simulink model "gtm_aeromodel"  (Simulink 7.2)
settings: Solver=ode45  StartTime=0.0  StopTime=10.0  RelTol=1e-3
undefined symbols (not defined in the file or in its folder): A_BLCG, A_BW, A_CW, A_FSCG, A_FSREF_in, A_SW, A_WLCG, A_WLREF, ALPHA0, bclowb, bclowbx_FMACH, bcmowb, bcmowbx_FHP, bcmowby_FMACH, cda, cdax_FLPDEF, cddr, cddrx_FMACH, cdo, cdox_FLPDEF, cdt1, cdt1x_mach, cdt2, cdt2x_mach, cdto, cdtox_mach, cdwb, cdwbx_FALPHA, cdwby_FMACH, clat, clatfr, clatfrx_FHP, clatfry_FMACH, clatx_mach, clawbfr, clawbfrx_FHP, clawbfry_FMACH, cldefr, cldefrx_FHP, cldefry_FMACH, cldtab, cldtabx_FMACH, clqwb, clqwbfr, clqwbfrx_FHP, clqwbfry_FMACH, clqwbx_mach, cltdd, cltddx_FHP, cltddy_FMACH, clwb, clwbtdd, clwbtddx_FHP, clwbtddy_FMACH, clwbx_FALPHA, clwby_FMACH, clwbzdd, clwbzddx_FHP, clwbzddy_FMACH, clzdd ... (+196)
libraries: model_lib x1
(part 4 of 10)

== system gtm_aeromodel/get aero forces and moments/AERODYNAMICS/Force  Coefficients/DRAG /bcddf ==
  flap : Inport  OutDataType=sfix(16)  OutScaling=2^0
  Logical Operator : Logic
  Logical Operator1 : Logic
  Product1 : Product  Inputs=3  OutDataType=sfix(16)  OutScaling=2^0  SaturateOnIntegerOverflow=on  RndMeth=Zero  InputSameDT=on  OutDataTypeStr=Inherit: Same as first input
  Product2 : Product  Inputs=3  OutDataType=sfix(16)  OutScaling=2^0  SaturateOnIntegerOverflow=on  RndMeth=Zero  InputSameDT=on  OutDataTypeStr=Inherit: Same as first input
  Relational Operator : RelationalOperator  Operator=>  InputSameDT=on
  Relational Operator1 : RelationalOperator  Operator=<=  InputSameDT=on
  Relational Operator2 : RelationalOperator  Operator=>  InputSameDT=on
  Relational Operator3 : RelationalOperator  Operator=<=  InputSameDT=on
  Relational Operator4 : RelationalOperator  Operator=>  InputSameDT=on
  Sum : Sum  Inputs=+++  OutDataType=sfix(16)  OutScaling=2^0  SaturateOnIntegerOverflow=on  InputSameDT=on  OutDataTypeStr=Inherit: Same as first input
  Sum2 : Sum  OutDataType=sfix(16)  OutScaling=2^0  SaturateOnIntegerOverflow=on  InputSameDT=on  OutDataTypeStr=Inherit: Same as first input
  Sum{3..5,8} (4 alike) : Sum  Inputs=-+  OutDataType=sfix(16)  OutScaling=2^0  SaturateOnIntegerOverflow=on  InputSameDT=on  OutDataTypeStr=Inherit: Same as first input
  Sum6 : Sum  OutDataType=sfix(16)  OutScaling=2^0  SaturateOnIntegerOverflow=on  InputSameDT=on  OutDataTypeStr=Inherit: Same as first input
  Switch5 : Switch  Threshold=0.5  SaturateOnIntegerOverflow=on  InputSameDT=on
  Switch6 : Switch  Threshold=0.5  SaturateOnIntegerOverflow=on  InputSameDT=on
  Switch7 : Switch  Threshold=0.5  SaturateOnIntegerOverflow=on  InputSameDT=on
  zero : Constant  Value=0  OutDataType=sfix(16)  OutScaling=2^0
  zero1 : Constant  Value=10  OutDataType=sfix(16)  OutScaling=2^0
  zero11 : Constant  Value=-0.01  OutDataType=sfix(16)  OutScaling=2^0
  zero12 : Constant  Value=-0.013  OutDataType=sfix(16)  OutScaling=2^0
  zero13 : Constant  Value=-0.0175  OutDataType=sfix(16)  OutScaling=2^0
  zero2 : Constant  Value=0  OutDataType=sfix(16)  OutScaling=2^0
  zero5 : Constant  Value=20  OutDataType=sfix(16)  OutScaling=2^0
  zero6 : Constant  Value=10  OutDataType=sfix(16)  OutScaling=2^0
  zero7 : Constant  Value=0.1  OutDataType=sfix(16)  OutScaling=2^0
  zero8 : Constant  Value=20  OutDataType=sfix(16)  OutScaling=2^0
  zero9 : Constant  Value=1/19  OutDataType=sfix(16)  OutScaling=2^0
  bcddf : Outport  OutDataType=sfix(16)  OutScaling=2^0  InitialOutput=0
  wires:
  Sum6/1 -> Switch7/1
  zero9/1 -> Product2/2
  Sum5/1 -> Product2/3
  zero8/1 -> Sum5/1
  Sum2/1 -> Switch6/1
  Switch7/1 -> Sum/3
  Switch6/1 -> Sum/2
  Switch5/1 -> Sum/1
  Relational Operator4/1 -> Switch7/2
  zero5/1 -> Relational Operator4/2, Relational Operator3/2
  Sum/1 -> bcddf/1
  zero2/1 -> Switch7/3, Switch6/3, Switch5/3
  Logical Operator1/1 -> Switch6/2
  Relational Operator3/1 -> Logical Operator1/2
  Relational Operator2/1 -> Logical Operator1/1
  zero1/1 -> Relational Operator2/2, Relational Operator1/2
  zero/1 -> Relational Operator/2
  Logical Operator/1 -> Switch5/2
  Relational Operator1/1 -> Logical Operator/2
  Relational Operator/1 -> Logical Operator/1
  Sum3/1 -> Product1/3
  zero6/1 -> Sum3/1
  flap/1 -> Sum5/2, Relational Operator4/1, Relational Operator3/1, Relational Operator2/1, Relational Operator1/1, Relational Operator/1, Sum3/2
  zero11/1 -> Switch5/1, Sum2/1, Sum4/1
  Sum4/1 -> Product1/1
  Product1/1 -> Sum2/2
  zero12/1 -> Sum4/2, Sum8/1, Sum6/1
  zero13/1 -> Sum8/2
  zero7/1 -> Product1/2
  Sum8/1 -> Product2/1
  Product2/1 -> Sum6/2

== system gtm_aeromodel/get aero forces and moments/AERODYNAMICS/Force  Coefficients/DRAG /bcdwb ==
  clwb : Inport  OutDataType=sfix(16)  OutScaling=2^0
  Product6 : Product  OutDataType=sfix(16)  OutScaling=2^0  SaturateOnIntegerOverflow=on  RndMeth=Zero  InputSameDT=on  OutDataTypeStr=Inherit: Same as first input
  bcwb : Sum  Inputs=-+  OutDataType=sfix(16)  OutScaling=2^0  SaturateOnIntegerOverflow=on  InputSameDT=on  OutDataTypeStr=Inherit: Same as first input
  bcwb_FC8 : Constant  Value=.003  OutDataType=sfix(16)  OutScaling=2^0
  bcwb_FC9 : Constant  Value=.023  OutDataType=sfix(16)  OutScaling=2^0
  bcdwb_ : Outport  OutDataType=sfix(16)  OutScaling=2^0  InitialOutput=0
  wires:
  bcwb_FC8/1 -> bcwb/1
  clwb/1 -> Product6/1
  bcwb_FC9/1 -> Product6/2
  Product6/1 -> bcwb/2
  bcwb/1 -> bcdwb_/1

== system gtm_aeromodel/get aero forces and moments/AERODYNAMICS/Force  Coefficients/LIFT/CLDETAB ==
  mach : Inport  OutDataType=sfix(16)  OutScaling=2^0
  eletab : Inport  Port=2  OutDataType=sfix(16)  OutScaling=2^0
  Product : Product  OutDataType=sfix(16)  OutScaling=2^0  SaturateOnIntegerOverflow=on  RndMeth=Zero  InputSameDT=on  OutDataTypeStr=Inherit: Same as first input
  cldetab_ : Subsystem  mask(1-D Table){z=cldtabx_FMACH, tab=cldtab}
      mask prompts: z "Z vector:"; tab "Table:"
      mask help: 1-D Table Look Up. Enter monotonic Z vector amd table. See the help for more info.
      mask Help: The Z vector must be monotonic.  Z indexes into the columns of the 1-D tables.   Table does not extrapolate beyound the break vectors
      mask Display: plot(@2)
  cldetab : Outport  OutDataType=sfix(16)  OutScaling=2^0  InitialOutput=0
  wires:
  cldetab_/1(Interp Value) -> Product/1
  Product/1 -> cldetab/1
  eletab/1 -> Product/2
  mach/1 -> cldetab_/1(Z)

== system gtm_aeromodel/get aero forces and moments/AERODYNAMICS/Force  Coefficients/LIFT/CLGE ==
  hob : Inport  OutDataType=sfix(16)  OutScaling=2^0
  alpha : Inport  Port=2  OutDataType=sfix(16)  OutScaling=2^0
  flap : Inport  Port=3  OutDataType=sfix(16)  OutScaling=2^0
  dclhob : Subsystem  mask(1-2-3 Table){@1=dclhobx_HOB, @2=dclhoby_FALPHA, @3=dclhobz_FLPDEF, @4=dclhob}
      mask prompts: @1 "X vector:"; @2 "Y vector:"; @3 "Z vector:"; @4 "Table:"
      mask help: 3-D Table Look Up. Enter monotonic X, Y and Z vectors and a matrix of 2-D tables. See the help for more info.
      mask init:
      | x=@1;y=@2;z=@3;tab=@4;
      mask Help: The X, Y and Z vectors must be monotonic.   The 3-D table is a horizontal concatenation of  2-D tables.  X  indexes into the columns of the 2-D tables & Y indexes into the rows of the 2-D tables.  Z indexes into the table levels (starting with the 1st 2-D table).   The input values are x, y and z respectively (e.g., top port = x).
      mask Display: plot([0 2 2 0 0],[0 0 2 2 0],[0 2 2.9 0.95 0],[2 2 2.7 2.7 2],[2 2.9 2.9 2 2],[0 0.85 2.7 2 0])
  cdge : Outport  OutDataType=sfix(16)  OutScaling=2^0  InitialOutput=0
  wires:
  dclhob/1(Interp Value) -> cdge/1
  hob/1 -> dclhob/1(X)
  alpha/1 -> dclhob/2(Y)
  flap/1 -> dclhob/3(Z)

== system gtm_aeromodel/get aero forces and moments/AERODYNAMICS/Force  Coefficients/LIFT/CLQWB ==
  note: fqsv=q*cbar/2vt
  mach : Inport  OutDataType=sfix(16)  OutScaling=2^0
  Q' : Inport  Port=2  OutDataType=sfix(16)  OutScaling=2^0
  flex : Inport  Port=3  OutDataType=sfix(16)  OutScaling=2^0
  altitude : Inport  Port=4  OutDataType=sfix(16)  OutScaling=2^0
  Product : Product  Inputs=3  OutDataType=sfix(16)  OutScaling=2^0  SaturateOnIntegerOverflow=on  RndMeth=Zero  InputSameDT=on  OutDataTypeStr=Inherit: Same as first input
  Switch5 : Switch  Threshold=0.5  SaturateOnIntegerOverflow=on  InputSameDT=on
  clqwb_ : Subsystem  mask(1-D Table){z=clqwbx_mach, tab=clqwb}
      mask prompts: z "Z vector:"; tab "Table:"
      mask help: 1-D Table Look Up. Enter monotonic Z vector amd table. See the help for more info.
      mask Help: The Z vector must be monotonic.  Z indexes into the columns of the 1-D tables.   Table does not extrapolate beyound the break vectors
      mask Display: plot(@2)
  clqwbfr : Subsystem  TreatAsAtomicUnit=on
  one : Constant  Value=1.0  OutDataType=sfix(16)  OutScaling=2^0
  clq : Outport  OutDataType=sfix(16)  OutScaling=2^0  InitialOutput=0
  wires:
  clqwb_/1(Interp Value) -> Product/1
  mach/1 -> clqwbfr/2(mach1), clqwb_/1(Z)
  altitude/1 -> clqwbfr/1(altitude)
  Switch5/1 -> Product/3
  one/1 -> Switch5/3
  flex/1 -> Switch5/2, clqwbfr/Enable
  clqwbfr/1(clqwbfr) -> Switch5/1
  Q'/1 -> Product/2
  Product/1 -> clq/1

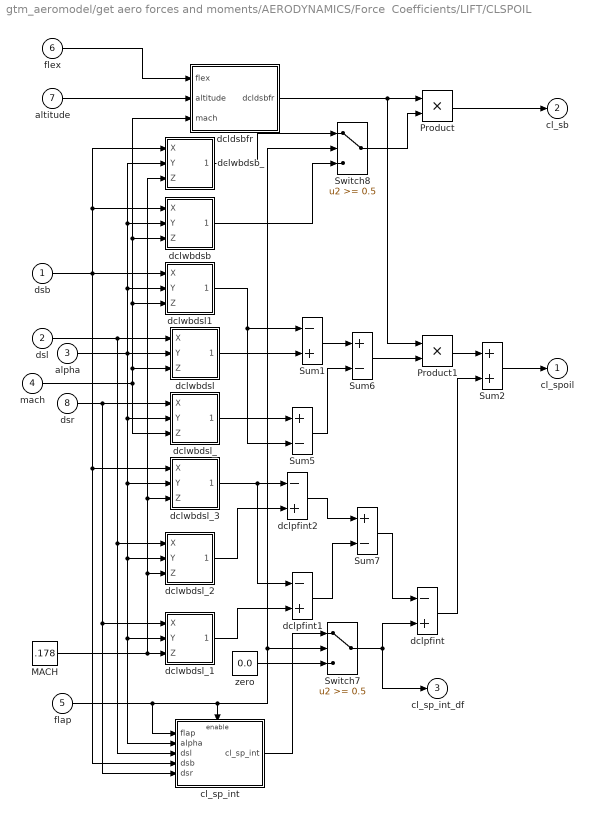
== system gtm_aeromodel/get aero forces and moments/AERODYNAMICS/Force  Coefficients/LIFT/CLSPOIL ==
  dsb : Inport  OutDataType=sfix(16)  OutScaling=2^0
  dsl : Inport  Port=2  OutDataType=sfix(16)  OutScaling=2^0
  alpha : Inport  Port=3  OutDataType=sfix(16)  OutScaling=2^0
  mach : Inport  Port=4  OutDataType=sfix(16)  OutScaling=2^0
  flap : Inport  Port=5  OutDataType=sfix(16)  OutScaling=2^0
  flex : Inport  Port=6  OutDataType=sfix(16)  OutScaling=2^0
  altitude : Inport  Port=7  OutDataType=sfix(16)  OutScaling=2^0
  dsr : Inport  Port=8  OutDataType=sfix(16)  OutScaling=2^0
  MACH : Constant  Value=.178  OutDataType=sfix(16)  OutScaling=2^0
  Product : Product  OutDataType=sfix(16)  OutScaling=2^0  SaturateOnIntegerOverflow=on  RndMeth=Zero  InputSameDT=on  OutDataTypeStr=Inherit: Same as first input
  Product1 : Product  OutDataType=sfix(16)  OutScaling=2^0  SaturateOnIntegerOverflow=on  RndMeth=Zero  InputSameDT=on  OutDataTypeStr=Inherit: Same as first input
  Sum1 : Sum  Inputs=-+  OutDataType=sfix(16)  OutScaling=2^0  SaturateOnIntegerOverflow=on  InputSameDT=on  OutDataTypeStr=Inherit: Same as first input
  Sum2 : Sum  OutDataType=sfix(16)  OutScaling=2^0  SaturateOnIntegerOverflow=on  InputSameDT=on  OutDataTypeStr=Inherit: Same as first input
  Sum5 : Sum  Inputs=+-  OutDataType=sfix(16)  OutScaling=2^0  SaturateOnIntegerOverflow=on  InputSameDT=on  OutDataTypeStr=Inherit: Same as first input
  Sum6 : Sum  Inputs=+-  OutDataType=sfix(16)  OutScaling=2^0  SaturateOnIntegerOverflow=on  InputSameDT=on  OutDataTypeStr=Inherit: Same as first input
  Sum7 : Sum  Inputs=+-  OutDataType=sfix(16)  OutScaling=2^0  SaturateOnIntegerOverflow=on  InputSameDT=on  OutDataTypeStr=Inherit: Same as first input
  Switch7 : Switch  Threshold=0.5  SaturateOnIntegerOverflow=on  InputSameDT=on
  Switch8 : Switch  Threshold=0.5  SaturateOnIntegerOverflow=on  InputSameDT=on
  cl_sp_int : Subsystem  TreatAsAtomicUnit=on
  dcldsbfr : Subsystem
  dclpfint : Sum  Inputs=-+  OutDataType=sfix(16)  OutScaling=2^0  SaturateOnIntegerOverflow=on  InputSameDT=on  OutDataTypeStr=Inherit: Same as first input
  dclpfint1 : Sum  Inputs=-+  OutDataType=sfix(16)  OutScaling=2^0  SaturateOnIntegerOverflow=on  InputSameDT=on  OutDataTypeStr=Inherit: Same as first input
  dclpfint2 : Sum  Inputs=-+  OutDataType=sfix(16)  OutScaling=2^0  SaturateOnIntegerOverflow=on  InputSameDT=on  OutDataTypeStr=Inherit: Same as first input
  dclwbdsb : Subsystem  mask(1-2-3 Table){@1=dclwbdsbx_DSB, @2=dclwbdsby_ALPHA, @3=dclwbdsbz_FMACH, @4=dclwbdsb}
      mask prompts: @1 "X vector:"; @2 "Y vector:"; @3 "Z vector:"; @4 "Table:"
      mask help: 3-D Table Look Up. Enter monotonic X, Y and Z vectors and a matrix of 2-D tables. See the help for more info.
      mask init:
      | x=@1;y=@2;z=@3;tab=@4;
      mask Help: The X, Y and Z vectors must be monotonic.   The 3-D table is a horizontal concatenation of  2-D tables.  X  indexes into the columns of the 2-D tables & Y indexes into the rows of the 2-D tables.  Z indexes into the table levels (starting with the 1st 2-D table).   The input values are x, y and z respectively (e.g., top port = x).
      mask Display: plot([0 2 2 0 0],[0 0 2 2 0],[0 2 2.9 0.95 0],[2 2 2.7 2.7 2],[2 2.9 2.9 2 2],[0 0.85 2.7 2 0])
  dclwbdsb_ : Subsystem  mask(1-2-3 Table){@1=dclwbdsbx_DSB, @2=dclwbdsby_ALPHA, @3=dclwbdsbz_FMACH, @4=dclwbdsb}
      mask prompts: @1 "X vector:"; @2 "Y vector:"; @3 "Z vector:"; @4 "Table:"
      mask help: 3-D Table Look Up. Enter monotonic X, Y and Z vectors and a matrix of 2-D tables. See the help for more info.
      mask init:
      | x=@1;y=@2;z=@3;tab=@4;
      mask Help: The X, Y and Z vectors must be monotonic.   The 3-D table is a horizontal concatenation of  2-D tables.  X  indexes into the columns of the 2-D tables & Y indexes into the rows of the 2-D tables.  Z indexes into the table levels (starting with the 1st 2-D table).   The input values are x, y and z respectively (e.g., top port = x).
      mask Display: plot([0 2 2 0 0],[0 0 2 2 0],[0 2 2.9 0.95 0],[2 2 2.7 2.7 2],[2 2.9 2.9 2 2],[0 0.85 2.7 2 0])
  dclwbdsl : Subsystem  mask(1-2-3 Table){@1=dclwbdslx_DSL, @2=dclwbdsly_FALPHA, @3=dclwbdslz_FMACH, @4=dclwbdsl}
      mask prompts: @1 "X vector:"; @2 "Y vector:"; @3 "Z vector:"; @4 "Table:"
      mask help: 3-D Table Look Up. Enter monotonic X, Y and Z vectors and a matrix of 2-D tables. See the help for more info.
      mask init:
      | x=@1;y=@2;z=@3;tab=@4;
      mask Help: The X, Y and Z vectors must be monotonic.   The 3-D table is a horizontal concatenation of  2-D tables.  X  indexes into the columns of the 2-D tables & Y indexes into the rows of the 2-D tables.  Z indexes into the table levels (starting with the 1st 2-D table).   The input values are x, y and z respectively (e.g., top port = x).
      mask Display: plot([0 2 2 0 0],[0 0 2 2 0],[0 2 2.9 0.95 0],[2 2 2.7 2.7 2],[2 2.9 2.9 2 2],[0 0.85 2.7 2 0])
  dclwbdsl1 : Subsystem  mask(1-2-3 Table){@1=dclwbdslx_DSL, @2=dclwbdsly_FALPHA, @3=dclwbdslz_FMACH, @4=dclwbdsl}
      mask prompts: @1 "X vector:"; @2 "Y vector:"; @3 "Z vector:"; @4 "Table:"
      mask help: 3-D Table Look Up. Enter monotonic X, Y and Z vectors and a matrix of 2-D tables. See the help for more info.
      mask init:
      | x=@1;y=@2;z=@3;tab=@4;
      mask Help: The X, Y and Z vectors must be monotonic.   The 3-D table is a horizontal concatenation of  2-D tables.  X  indexes into the columns of the 2-D tables & Y indexes into the rows of the 2-D tables.  Z indexes into the table levels (starting with the 1st 2-D table).   The input values are x, y and z respectively (e.g., top port = x).
      mask Display: plot([0 2 2 0 0],[0 0 2 2 0],[0 2 2.9 0.95 0],[2 2 2.7 2.7 2],[2 2.9 2.9 2 2],[0 0.85 2.7 2 0])
  dclwbdsl_ : Subsystem  mask(1-2-3 Table){@1=dclwbdslx_DSL, @2=dclwbdsly_FALPHA, @3=dclwbdslz_FMACH, @4=dclwbdsl}
      mask prompts: @1 "X vector:"; @2 "Y vector:"; @3 "Z vector:"; @4 "Table:"
      mask help: 3-D Table Look Up. Enter monotonic X, Y and Z vectors and a matrix of 2-D tables. See the help for more info.
      mask init:
      | x=@1;y=@2;z=@3;tab=@4;
      mask Help: The X, Y and Z vectors must be monotonic.   The 3-D table is a horizontal concatenation of  2-D tables.  X  indexes into the columns of the 2-D tables & Y indexes into the rows of the 2-D tables.  Z indexes into the table levels (starting with the 1st 2-D table).   The input values are x, y and z respectively (e.g., top port = x).
      mask Display: plot([0 2 2 0 0],[0 0 2 2 0],[0 2 2.9 0.95 0],[2 2 2.7 2.7 2],[2 2.9 2.9 2 2],[0 0.85 2.7 2 0])
  dclwbdsl_1 : Subsystem  mask(1-2-3 Table){@1=dclwbdslx_DSL, @2=dclwbdsly_FALPHA, @3=dclwbdslz_FMACH, @4=dclwbdsl}
      mask prompts: @1 "X vector:"; @2 "Y vector:"; @3 "Z vector:"; @4 "Table:"
      mask help: 3-D Table Look Up. Enter monotonic X, Y and Z vectors and a matrix of 2-D tables. See the help for more info.
      mask init:
      | x=@1;y=@2;z=@3;tab=@4;
      mask Help: The X, Y and Z vectors must be monotonic.   The 3-D table is a horizontal concatenation of  2-D tables.  X  indexes into the columns of the 2-D tables & Y indexes into the rows of the 2-D tables.  Z indexes into the table levels (starting with the 1st 2-D table).   The input values are x, y and z respectively (e.g., top port = x).
      mask Display: plot([0 2 2 0 0],[0 0 2 2 0],[0 2 2.9 0.95 0],[2 2 2.7 2.7 2],[2 2.9 2.9 2 2],[0 0.85 2.7 2 0])
  dclwbdsl_2 : Subsystem  mask(1-2-3 Table){@1=dclwbdslx_DSL, @2=dclwbdsly_FALPHA, @3=dclwbdslz_FMACH, @4=dclwbdsl}
      mask prompts: @1 "X vector:"; @2 "Y vector:"; @3 "Z vector:"; @4 "Table:"
      mask help: 3-D Table Look Up. Enter monotonic X, Y and Z vectors and a matrix of 2-D tables. See the help for more info.
      mask init:
      | x=@1;y=@2;z=@3;tab=@4;
      mask Help: The X, Y and Z vectors must be monotonic.   The 3-D table is a horizontal concatenation of  2-D tables.  X  indexes into the columns of the 2-D tables & Y indexes into the rows of the 2-D tables.  Z indexes into the table levels (starting with the 1st 2-D table).   The input values are x, y and z respectively (e.g., top port = x).
      mask Display: plot([0 2 2 0 0],[0 0 2 2 0],[0 2 2.9 0.95 0],[2 2 2.7 2.7 2],[2 2.9 2.9 2 2],[0 0.85 2.7 2 0])
  dclwbdsl_3 : Subsystem  mask(1-2-3 Table){@1=dclwbdslx_DSL, @2=dclwbdsly_FALPHA, @3=dclwbdslz_FMACH, @4=dclwbdsl}
      mask prompts: @1 "X vector:"; @2 "Y vector:"; @3 "Z vector:"; @4 "Table:"
      mask help: 3-D Table Look Up. Enter monotonic X, Y and Z vectors and a matrix of 2-D tables. See the help for more info.
      mask init:
      | x=@1;y=@2;z=@3;tab=@4;
      mask Help: The X, Y and Z vectors must be monotonic.   The 3-D table is a horizontal concatenation of  2-D tables.  X  indexes into the columns of the 2-D tables & Y indexes into the rows of the 2-D tables.  Z indexes into the table levels (starting with the 1st 2-D table).   The input values are x, y and z respectively (e.g., top port = x).
      mask Display: plot([0 2 2 0 0],[0 0 2 2 0],[0 2 2.9 0.95 0],[2 2 2.7 2.7 2],[2 2.9 2.9 2 2],[0 0.85 2.7 2 0])
  zero : Constant  Value=0.0  OutDataType=sfix(16)  OutScaling=2^0
  cl_spoil : Outport  OutDataType=sfix(16)  OutScaling=2^0  InitialOutput=0
  cl_sb : Outport  Port=2  OutDataType=sfix(16)  OutScaling=2^0  InitialOutput=0
  cl_sp_int_df : Outport  Port=3  OutDataType=sfix(16)  OutScaling=2^0  InitialOutput=0
  wires:
  flex/1 -> dcldsbfr/1(flex)
  dclwbdsb_/1(Interp Value) -> Switch8/1
  dclwbdsb/1(Interp Value) -> Switch8/3
  dclwbdsl1/1(Interp Value) -> Sum5/2, Sum1/1
  MACH/1 -> dclwbdsb_/3(Z), dclwbdsl_3/3(Z), dclwbdsl_2/3(Z), dclwbdsl_1/3(Z)
  Sum7/1 -> dclpfint/1
  dclpfint1/1 -> Sum7/2
  dclpfint2/1 -> Sum7/1
  dclwbdsl_2/1(Interp Value) -> dclpfint2/2
  dclwbdsl_3/1(Interp Value) -> dclpfint2/1, dclpfint1/1
  dclwbdsl_1/1(Interp Value) -> dclpfint1/2
  dsr/1 -> cl_sp_int/5(dsr), dclwbdsl_1/1(X), dclwbdsl_/1(X)
  mach/1 -> dclwbdsl_/3(Z), dclwbdsb/3(Z), dcldsbfr/3(mach), dclwbdsl1/3(Z), dclwbdsl/3(Z)
  dclwbdsl/1(Interp Value) -> Sum1/2
  alpha/1 -> dclwbdsl_2/2(Y), dclwbdsl_1/2(Y), cl_sp_int/2(alpha), dclwbdsl_3/2(Y), dclwbdsl_/2(Y), dclwbdsl/2(Y), dclwbdsl1/2(Y), dclwbdsb/2(Y), dclwbdsb_/2(Y)
  dsl/1 -> dclwbdsl_2/1(X), cl_sp_int/3(dsl), dclwbdsl/1(X)
  Sum6/1 -> Product1/2
  Sum5/1 -> Sum6/2
  Sum1/1 -> Sum6/1
  dclwbdsl_/1(Interp Value) -> Sum5/1
  dclpfint/1 -> Sum2/2
  Product1/1 -> Sum2/1
  Sum2/1 -> cl_spoil/1
  flap/1 -> cl_sp_int/1(flap), Switch8/2, Switch7/2, cl_sp_int/Enable
  cl_sp_int/1(cl_sp_int) -> Switch7/1
  zero/1 -> Switch7/3
  dsb/1 -> dclwbdsb_/1(X), dclwbdsb/1(X), dclwbdsl_3/1(X), cl_sp_int/4(dsb), dclwbdsl1/1(X)
  dcldsbfr/1(dcldsbfr) -> Product1/1, Product/1
  Product/1 -> cl_sb/1
  Switch8/1 -> Product/2
  altitude/1 -> dcldsbfr/2(altitude)
  Switch7/1 -> dclpfint/2, cl_sp_int_df/1

== system gtm_aeromodel/get aero forces and moments/AERODYNAMICS/Force  Coefficients/LIFT/CLTP ==
  mach : Inport  OutDataType=sfix(16)  OutScaling=2^0
  alphat : Inport  Port=2  OutDataType=sfix(16)  OutScaling=2^0
  altitude : Inport  Port=3  OutDataType=sfix(16)  OutScaling=2^0
  norm acc g's : Inport  Port=4  OutDataType=sfix(16)  OutScaling=2^0
  qdot : Inport  Port=5  OutDataType=sfix(16)  OutScaling=2^0
  flex : Inport  Port=6  OutDataType=sfix(16)  OutScaling=2^0
  Product1 : Product  OutDataType=sfix(16)  OutScaling=2^0  SaturateOnIntegerOverflow=on  RndMeth=Zero  InputSameDT=on  OutDataTypeStr=Inherit: Same as first input
  Product2 : Product  OutDataType=sfix(16)  OutScaling=2^0  SaturateOnIntegerOverflow=on  RndMeth=Zero  InputSameDT=on  OutDataTypeStr=Inherit: Same as first input
  Switch6 : Switch  Threshold=0.5  SaturateOnIntegerOverflow=on  InputSameDT=on
  Switch7 : Switch  Threshold=0.5  SaturateOnIntegerOverflow=on  InputSameDT=on
  clat : Subsystem  mask(1-D Table){z=clatx_mach, tab=clat}
      mask prompts: z "Z vector:"; tab "Table:"
      mask help: 1-D Table Look Up. Enter monotonic Z vector amd table. See the help for more info.
      mask Help: The Z vector must be monotonic.  Z indexes into the columns of the 1-D tables.   Table does not extrapolate beyound the break vectors
      mask Display: plot(@2)
  cltailflx : Subsystem  TreatAsAtomicUnit=on
  one : Constant  OutDataType=sfix(16)  OutScaling=2^0
  zero : Constant  Value=0.0  OutDataType=sfix(16)  OutScaling=2^0
  cltp : Outport  OutDataType=sfix(16)  OutScaling=2^0  InitialOutput=0
  cltfr : Outport  Port=2  OutDataType=sfix(16)  OutScaling=2^0  InitialOutput=0
  wires:
  clat/1(Interp Value) -> Product1/1
  Switch7/1 -> Product1/2
  Product1/1 -> Product2/1
  alphat/1 -> Product2/2
  Product2/1 -> cltp/1
  one/1 -> Switch7/3
  cltailflx/2(clatfr) -> Switch7/1
  altitude/1 -> cltailflx/1(altitude)
  qdot/1 -> cltailflx/4(qdot)
  norm acc g's/1 -> cltailflx/3(norm acc g's)
  Switch6/1 -> cltfr/1
  cltailflx/1(cltflx) -> Switch6/1
  flex/1 -> Switch7/2, cltailflx/Enable, Switch6/2
  zero/1 -> Switch6/3
  mach/1 -> cltailflx/2(Mach), clat/1(Z)

== system gtm_aeromodel/get aero forces and moments/AERODYNAMICS/Force  Coefficients/LIFT/CLWB ==
  alpha : Inport  OutDataType=sfix(16)  OutScaling=2^0
  mach : Inport  Port=2  OutDataType=sfix(16)  OutScaling=2^0
  flap : Inport  Port=3  OutDataType=sfix(16)  OutScaling=2^0
  flex : Inport  Port=4  OutDataType=sfix(16)  OutScaling=2^0
  altitude : Inport  Port=5  OutDataType=sfix(16)  OutScaling=2^0
  qdyn : Inport  Port=6  OutDataType=sfix(16)  OutScaling=2^0
  norm acc g's : Inport  Port=7  OutDataType=sfix(16)  OutScaling=2^0
  qdot : Inport  Port=8  OutDataType=sfix(16)  OutScaling=2^0
  dsb : Inport  Port=9  OutDataType=sfix(16)  OutScaling=2^0
  CLWBFLEX : Subsystem  TreatAsAtomicUnit=on
  Product1 : Product  OutDataType=sfix(16)  OutScaling=2^0  SaturateOnIntegerOverflow=on  RndMeth=Zero  InputSameDT=on  OutDataTypeStr=Inherit: Same as first input
  Sum : Sum  OutDataType=sfix(16)  OutScaling=2^0  SaturateOnIntegerOverflow=on  InputSameDT=on  OutDataTypeStr=Inherit: Same as first input
  Sum2 : Sum  Inputs=+-  OutDataType=sfix(16)  OutScaling=2^0  SaturateOnIntegerOverflow=on  InputSameDT=on  OutDataTypeStr=Inherit: Same as first input
  Sum4 : Sum  OutDataType=sfix(16)  OutScaling=2^0  SaturateOnIntegerOverflow=on  InputSameDT=on  OutDataTypeStr=Inherit: Same as first input
  Switch{5..6,8,10} (4 alike) : Switch  Threshold=0.5  SaturateOnIntegerOverflow=on  InputSameDT=on
  cl_flap_ : Subsystem  TreatAsAtomicUnit=on
  clwb_ : Subsystem  mask(2-D Table){y=clwbx_FALPHA, z=clwby_FMACH, tab=clwb}
      mask prompts: y "Y vector:"; z "Z vector:"; tab "Table:"
      mask help: 2-D Table Look Up. Enter monotonic Y and Z vectors and a matrix of 2-D tables. See the help for more info.
      mask Help: The Y and Z vectors must be monotonic.  Y  indexes into the columns of the 2-D table & Z indexes into the rows of the 2-D tables.   The input values are y and z respectively (e.g., top port = y).
      mask Display: plot(-10,-10,110,110,[90,50,10],[90,40,30],[90,50,10],[50,26,20],[90,50,10],[22,13,10])
  clwb_zero : Subsystem  mask(2-D Table){y=clwbx_FALPHA, z=clwby_FMACH, tab=clwb}
      mask prompts: y "Y vector:"; z "Z vector:"; tab "Table:"
      mask help: 2-D Table Look Up. Enter monotonic Y and Z vectors and a matrix of 2-D tables. See the help for more info.
      mask Help: The Y and Z vectors must be monotonic.  Y  indexes into the columns of the 2-D table & Z indexes into the rows of the 2-D tables.   The input values are y and z respectively (e.g., top port = y).
      mask Display: plot(-10,-10,110,110,[90,50,10],[90,40,30],[90,50,10],[50,26,20],[90,50,10],[22,13,10])
  constant1 : Constant  Value=0.0  OutDataType=sfix(16)  OutScaling=2^0
  constant3 : Constant  Value=1.0  OutDataType=sfix(16)  OutScaling=2^0
  zero : Constant  Value=0.0  OutDataType=sfix(16)  OutScaling=2^0
  zero_ : Constant  Value=0.0  OutDataType=sfix(16)  OutScaling=2^0
  clwb : Outport  OutDataType=sfix(16)  OutScaling=2^0  InitialOutput=0
  cl_flap : Outport  Port=2  OutDataType=sfix(16)  OutScaling=2^0  InitialOutput=0
  dclsbfint : Outport  Port=3  OutDataType=sfix(16)  OutScaling=2^0  InitialOutput=0
  cl_flx : Outport  Port=4  OutDataType=sfix(16)  OutScaling=2^0  InitialOutput=0
  wires:
  CLWBFLEX/2(cl_flx) -> cl_flx/1
  CLWBFLEX/1(clawbfr) -> Switch8/1
  constant3/1 -> Switch8/3
  CLWBFLEX/3(fdclowb) -> Switch6/1
  Product1/1 -> Sum/2
  Sum4/1 -> Sum/1
  Switch10/1 -> dclsbfint/1
  cl_flap_/2(dclsbfint) -> Switch10/1
  dsb/1 -> cl_flap_/5(dsb)
  Switch8/1 -> Product1/2
  flex/1 -> cl_flap_/4(flex), Switch8/2, Switch6/2, CLWBFLEX/Enable
  qdot/1 -> CLWBFLEX/4(qdot)
  norm acc g's/1 -> CLWBFLEX/3(norm acc g's)
  clwb_zero/1(Interp Value) -> Sum2/2, Sum4/2
  zero/1 -> clwb_zero/1(Y)
  altitude/1 -> CLWBFLEX/1(altitude)
  constant1/1 -> Switch6/3
  qdyn/1 -> cl_flap_/3(qdyn)
  alpha/1 -> cl_flap_/2(alpha), clwb_/1(Y)
  mach/1 -> clwb_zero/2(Z), CLWBFLEX/2(Mach), clwb_/2(Z)
  cl_flap_/1(cl_flap) -> Switch5/1
  flap/1 -> cl_flap_/1(flap), cl_flap_/Enable, Switch5/2, Switch10/2
  zero_/1 -> Switch5/3, Switch10/3
  Switch6/1 -> Sum4/1
  clwb_/1(Interp Value) -> Sum2/1
  Sum2/1 -> Product1/1
  Switch5/1 -> cl_flap/1
  Sum/1 -> clwb/1

== system gtm_aeromodel/get aero forces and moments/AERODYNAMICS/Force  Coefficients/LIFT/DCLDE ==
  elev : Inport  OutDataType=sfix(16)  OutScaling=2^0
  alphat : Inport  Port=2  OutDataType=sfix(16)  OutScaling=2^0
  mach : Inport  Port=3  OutDataType=sfix(16)  OutScaling=2^0
  flex : Inport  Port=4  OutDataType=sfix(16)  OutScaling=2^0
  altitude : Inport  Port=5  OutDataType=sfix(16)  OutScaling=2^0
  Product : Product  OutDataType=sfix(16)  OutScaling=2^0  SaturateOnIntegerOverflow=on  RndMeth=Zero  InputSameDT=on  OutDataTypeStr=Inherit: Same as first input
  Switch5 : Switch  Threshold=0.5  SaturateOnIntegerOverflow=on  InputSameDT=on
  cldefr : Subsystem  TreatAsAtomicUnit=on
  constant3 : Constant  Value=1.0  OutDataType=sfix(16)  OutScaling=2^0
  dclde_ : Subsystem  mask(1-2-3 Table){@1=dcldex_FELE, @2=dcldey_ALPHAT, @3=dcldez_FMACH, @4=dclde}
      mask prompts: @1 "X vector:"; @2 "Y vector:"; @3 "Z vector:"; @4 "Table:"
      mask help: 3-D Table Look Up. Enter monotonic X, Y and Z vectors and a matrix of 2-D tables. See the help for more info.
      mask init:
      | x=@1;y=@2;z=@3;tab=@4;
      mask Help: The X, Y and Z vectors must be monotonic.   The 3-D table is a horizontal concatenation of  2-D tables.  X  indexes into the columns of the 2-D tables & Y indexes into the rows of the 2-D tables.  Z indexes into the table levels (starting with the 1st 2-D table).   The input values are x, y and z respectively (e.g., top port = x).
      mask Display: plot([0 2 2 0 0],[0 0 2 2 0],[0 2 2.9 0.95 0],[2 2 2.7 2.7 2],[2 2.9 2.9 2 2],[0 0.85 2.7 2 0])
  dclde : Outport  OutDataType=sfix(16)  OutScaling=2^0  InitialOutput=0
  wires:
  constant3/1 -> Switch5/3
  Switch5/1 -> Product/2
  Product/1 -> dclde/1
  dclde_/1(Interp Value) -> Product/1
  flex/1 -> Switch5/2, cldefr/Enable
  cldefr/1(cldefr) -> Switch5/1
  altitude/1 -> cldefr/1(altitude)
  mach/1 -> cldefr/2(mach), dclde_/3(Z)
  elev/1 -> dclde_/1(X)
  alphat/1 -> dclde_/2(Y)

== system gtm_aeromodel/get aero forces and moments/AERODYNAMICS/Force  Coefficients/LIFT/bcldf ==
  flap : Inport  OutDataType=sfix(16)  OutScaling=2^0
  alpha : Inport  Port=2  OutDataType=sfix(16)  OutScaling=2^0
  Logical Operator : Logic  AllPortsSameDT=off
  Logical Operator1 : Logic
  Product : Product  OutDataType=sfix(16)  OutScaling=2^0  SaturateOnIntegerOverflow=on  RndMeth=Zero  InputSameDT=on  OutDataTypeStr=Inherit: Same as first input
  Product1 : Product  Inputs=3  OutDataType=sfix(16)  OutScaling=2^0  SaturateOnIntegerOverflow=on  RndMeth=Zero  InputSameDT=on  OutDataTypeStr=Inherit: Same as first input
  Product2 : Product  Inputs=3  OutDataType=sfix(16)  OutScaling=2^0  SaturateOnIntegerOverflow=on  RndMeth=Zero  InputSameDT=on  OutDataTypeStr=Inherit: Same as first input
  Relational Operator1 : RelationalOperator  Operator=<=  InputSameDT=on
  Relational Operator2 : RelationalOperator  Operator=>  InputSameDT=on
  Relational Operator3 : RelationalOperator  Operator=<=  InputSameDT=on
  Relational Operator4 : RelationalOperator  Operator=>  InputSameDT=on
  Sum : Sum  Inputs=+++  OutDataType=sfix(16)  OutScaling=2^0  SaturateOnIntegerOverflow=on  InputSameDT=on  OutDataTypeStr=Inherit: Same as first input
  Sum{1,3..5,7} (5 alike) : Sum  Inputs=-+  OutDataType=sfix(16)  OutScaling=2^0  SaturateOnIntegerOverflow=on  InputSameDT=on  OutDataTypeStr=Inherit: Same as first input
  Sum2 : Sum  Inputs=++-  OutDataType=sfix(16)  OutScaling=2^0  SaturateOnIntegerOverflow=on  InputSameDT=on  OutDataTypeStr=Inherit: Same as first input
  Sum6 : Sum  Inputs=++-  OutDataType=sfix(16)  OutScaling=2^0  SaturateOnIntegerOverflow=on  InputSameDT=on  OutDataTypeStr=Inherit: Same as first input
  Switch5 : Switch  Threshold=0.5  SaturateOnIntegerOverflow=on  InputSameDT=on
  Switch6 : Switch  Threshold=0.5  SaturateOnIntegerOverflow=on  InputSameDT=on
  Switch7 : Switch  Threshold=0.5  SaturateOnIntegerOverflow=on  InputSameDT=on
  zero : Constant  Value=0  OutDataType=sfix(16)  OutScaling=2^0
  zero1 : Constant  Value=10  OutDataType=sfix(16)  OutScaling=2^0
  zero10 : Constant  Value=.12  OutDataType=sfix(16)  OutScaling=2^0
  zero2 : Constant  Value=0  OutDataType=sfix(16)  OutScaling=2^0
  zero3 : Constant  Value=.0065  OutDataType=sfix(16)  OutScaling=2^0
  zero4 : Constant  Value=.065  OutDataType=sfix(16)  OutScaling=2^0
  zero5 : Constant  Value=20  OutDataType=sfix(16)  OutScaling=2^0
  zero6 : Constant  Value=10  OutDataType=sfix(16)  OutScaling=2^0
  zero7 : Constant  Value=0.1  OutDataType=sfix(16)  OutScaling=2^0
  zero8 : Constant  Value=20  OutDataType=sfix(16)  OutScaling=2^0
  zero9 : Constant  Value=1/19  OutDataType=sfix(16)  OutScaling=2^0
  bcldf : Outport  OutDataType=sfix(16)  OutScaling=2^0  InitialOutput=0
  wires:
  zero/1 -> Logical Operator/1
  alpha/1 -> Product/2
  zero3/1 -> Product/1
  Product/1 -> Sum1/2, Sum2/2, Sum6/2
  flap/1 -> Sum3/2, Relational Operator1/1, Relational Operator2/1, Relational Operator3/1, Relational Operator4/1, Sum5/2
  zero6/1 -> Sum3/1
  zero7/1 -> Sum4/2, Product1/2, Sum7/1, Sum6/1
  zero4/1 -> Sum1/1, Sum4/1, Sum2/1
  Sum3/1 -> Product1/3
  Sum4/1 -> Product1/1
  Product1/1 -> Sum2/3
  Relational Operator1/1 -> Logical Operator/2
  Logical Operator/1 -> Switch5/2
  Sum1/1 -> Switch5/1
  zero1/1 -> Relational Operator1/2, Relational Operator2/2
  Relational Operator2/1 -> Logical Operator1/1
  Relational Operator3/1 -> Logical Operator1/2
  Logical Operator1/1 -> Switch6/2
  zero2/1 -> Switch5/3, Switch6/3, Switch7/3
  Sum/1 -> bcldf/1
  zero5/1 -> Relational Operator3/2, Relational Operator4/2
  Relational Operator4/1 -> Switch7/2
  Switch5/1 -> Sum/1
  Switch6/1 -> Sum/2
  Switch7/1 -> Sum/3
  Sum2/1 -> Switch6/1
  zero8/1 -> Sum5/1
  Sum5/1 -> Product2/3
  zero9/1 -> Product2/2
  zero10/1 -> Sum7/2
  Sum7/1 -> Product2/1
  Product2/1 -> Sum6/3
  Sum6/1 -> Switch7/1

== system gtm_aeromodel/get aero forces and moments/AERODYNAMICS/Force  Coefficients/LIFT/bclowb ==
  mach : Inport  OutDataType=sfix(16)  OutScaling=2^0
  bclowb_ : Subsystem  mask(1-D Table){z=bclowbx_FMACH, tab=bclowb}
      mask prompts: z "Z vector:"; tab "Table:"
      mask help: 1-D Table Look Up. Enter monotonic Z vector amd table. See the help for more info.
      mask Help: The Z vector must be monotonic.  Z indexes into the columns of the 1-D tables.   Table does not extrapolate beyound the break vectors
      mask Display: plot(@2)
  bclowb : Outport  OutDataType=sfix(16)  OutScaling=2^0  InitialOutput=0
  wires:
  bclowb_/1(Interp Value) -> bclowb/1
  mach/1 -> bclowb_/1(Z)

== system gtm_aeromodel/get aero forces and moments/AERODYNAMICS/Force  Coefficients/SIDE/CYBWB ==
  alpha : Inport  OutDataType=sfix(16)  OutScaling=2^0
  mach : Inport  Port=2  OutDataType=sfix(16)  OutScaling=2^0
  flap : Inport  Port=3  OutDataType=sfix(16)  OutScaling=2^0
  flex : Inport  Port=4  OutDataType=sfix(16)  OutScaling=2^0
  altitude : Inport  Port=5  OutDataType=sfix(16)  OutScaling=2^0
  CYWBFLEX : Subsystem  TreatAsAtomicUnit=on
  Sum : Sum  OutDataType=sfix(16)  OutScaling=2^0  SaturateOnIntegerOverflow=on  InputSameDT=on  OutDataTypeStr=Inherit: Same as first input
  Switch5 : Switch  Threshold=0.1  SaturateOnIntegerOverflow=on  InputSameDT=on
  constant : Constant  Value=0.0  OutDataType=sfix(16)  OutScaling=2^0
  cy_flap_ : Subsystem  TreatAsAtomicUnit=on
  cybwb : Subsystem  mask(2-D Table){y=cybwbx_FMACH, z=cybwby_FALPHA, tab=cybwb}
      mask prompts: y "Y vector:"; z "Z vector:"; tab "Table:"
      mask help: 2-D Table Look Up. Enter monotonic Y and Z vectors and a matrix of 2-D tables. See the help for more info.
      mask Help: The Y and Z vectors must be monotonic.  Y  indexes into the columns of the 2-D table & Z indexes into the rows of the 2-D tables.   The input values are y and z respectively (e.g., top port = y).
      mask Display: plot(-10,-10,110,110,[90,50,10],[90,40,30],[90,50,10],[50,26,20],[90,50,10],[22,13,10])
  cywb+fl : Outport  OutDataType=sfix(16)  OutScaling=2^0  InitialOutput=0
  cybfr : Outport  Port=2  OutDataType=sfix(16)  OutScaling=2^0  InitialOutput=0
  wires:
  mach/1 -> cybwb/1(Y), CYWBFLEX/2(Mach)
  alpha/1 -> cybwb/2(Z), cy_flap_/2(alpha)
  flap/1 -> cy_flap_/Enable, Switch5/2, cy_flap_/1(flap)
  cy_flap_/1(cy_flap) -> Switch5/1
  altitude/1 -> CYWBFLEX/1(altitude)
  constant/1 -> Switch5/3
  flex/1 -> CYWBFLEX/Enable
  Sum/1 -> cywb+fl/1
  CYWBFLEX/1(cybfr) -> cybfr/1
  Switch5/1 -> Sum/1
  cybwb/1(Interp Value) -> Sum/2

== system gtm_aeromodel/get aero forces and moments/AERODYNAMICS/Force  Coefficients/SIDE/CYGEAR ==
  flap : Inport  OutDataType=sfix(16)  OutScaling=2^0
  alpha : Inport  Port=2  OutDataType=sfix(16)  OutScaling=2^0
  gear : Inport  Port=3  OutDataType=sfix(16)  OutScaling=2^0
  beta : Inport  Port=4  OutDataType=sfix(16)  OutScaling=2^0
  Product : Product  OutDataType=sfix(16)  OutScaling=2^0  SaturateOnIntegerOverflow=on  RndMeth=Zero  InputSameDT=on  OutDataTypeStr=Inherit: Same as first input
  Product1 : Product  OutDataType=sfix(16)  OutScaling=2^0  SaturateOnIntegerOverflow=on  RndMeth=Zero  InputSameDT=on  OutDataTypeStr=Inherit: Same as first input
  Sum1 : Sum  OutDataType=sfix(16)  OutScaling=2^0  SaturateOnIntegerOverflow=on  InputSameDT=on  OutDataTypeStr=Inherit: Same as first input
  Switch6 : Switch  Threshold=0.5  SaturateOnIntegerOverflow=on  InputSameDT=on
  constant1 : Constant  Value=0.0  OutDataType=sfix(16)  OutScaling=2^0
  dcyba : Subsystem  mask(1-D Table){z=dcybax_FLPDEF, tab=dcyba}
      mask prompts: z "Z vector:"; tab "Table:"
      mask help: 1-D Table Look Up. Enter monotonic Z vector amd table. See the help for more info.
      mask Help: The Z vector must be monotonic.  Z indexes into the columns of the 1-D tables.   Table does not extrapolate beyound the break vectors
      mask Display: plot(@2)
  dcybo : Subsystem  mask(1-D Table){z=dcybox_FLPDEF, tab=dcybo}
      mask prompts: z "Z vector:"; tab "Table:"
      mask help: 1-D Table Look Up. Enter monotonic Z vector amd table. See the help for more info.
      mask Help: The Z vector must be monotonic.  Z indexes into the columns of the 1-D tables.   Table does not extrapolate beyound the break vectors
      mask Display: plot(@2)
  cdg : Outport  OutDataType=sfix(16)  OutScaling=2^0  InitialOutput=0
  wires:
  Product1/1 -> Switch6/1
  beta/1 -> Product1/1
  Sum1/1 -> Product1/2
  Switch6/1 -> cdg/1
  constant1/1 -> Switch6/3
  gear/1 -> Switch6/2
  dcybo/1(Interp Value) -> Sum1/1
  Product/1 -> Sum1/2
  alpha/1 -> Product/2
  dcyba/1(Interp Value) -> Product/1
  flap/1 -> dcyba/1(Z), dcybo/1(Z)

== system gtm_aeromodel/get aero forces and moments/AERODYNAMICS/Force  Coefficients/SIDE/CYP ==
  mach : Inport  OutDataType=sfix(16)  OutScaling=2^0
  alpha : Inport  Port=2  OutDataType=sfix(16)  OutScaling=2^0
  altitude : Inport  Port=3  OutDataType=sfix(16)  OutScaling=2^0
  flex : Inport  Port=4  OutDataType=sfix(16)  OutScaling=2^0
  p_prime : Inport  Port=5  OutDataType=sfix(16)  OutScaling=2^0
  CYPFLEX : Subsystem  TreatAsAtomicUnit=on
  Fcn28 : Fcn  Expr=1/u
  Product2 : Product  Inputs=5  OutDataType=sfix(16)  OutScaling=2^0  SaturateOnIntegerOverflow=on  RndMeth=Zero  InputSameDT=on  OutDataTypeStr=Inherit: Same as first input
  Switch7 : Switch  Threshold=0.5  SaturateOnIntegerOverflow=on  InputSameDT=on
  constant : Constant  OutDataType=sfix(16)  OutScaling=2^0
  constant2 : Constant  Value=2  OutDataType=sfix(16)  OutScaling=2^0
  constant3 : Constant  Value=constants.r2d  OutDataType=sfix(16)  OutScaling=2^0
  cyptail : Product  OutDataType=sfix(16)  OutScaling=2^0  SaturateOnIntegerOverflow=on  RndMeth=Zero  InputSameDT=on  OutDataTypeStr=Inherit: Same as first input
  cyptot : Sum  Inputs=|++  OutDataType=sfix(16)  OutScaling=2^0  SaturateOnIntegerOverflow=on  InputSameDT=on  OutDataTypeStr=Inherit: Same as first input
  cypwb : Product  OutDataType=sfix(16)  OutScaling=2^0  SaturateOnIntegerOverflow=on  RndMeth=Zero  InputSameDT=on  OutDataTypeStr=Inherit: Same as first input
  dcyrt : Product  OutDataType=sfix(16)  OutScaling=2^0  SaturateOnIntegerOverflow=on  RndMeth=Zero  InputSameDT=on  OutDataTypeStr=Inherit: Same as first input
  rcrbvt : Subsystem  mask(2-D Table){y=crbvtx_FMACH, z=crbvty_FALPHA, tab=crbvt}
      mask prompts: y "Y vector:"; z "Z vector:"; tab "Table:"
      mask help: 2-D Table Look Up. Enter monotonic Y and Z vectors and a matrix of 2-D tables. See the help for more info.
      mask Help: The Y and Z vectors must be monotonic.  Y  indexes into the columns of the 2-D table & Z indexes into the rows of the 2-D tables.   The input values are y and z respectively (e.g., top port = y).
      mask Display: plot(-10,-10,110,110,[90,50,10],[90,40,30],[90,50,10],[50,26,20],[90,50,10],[22,13,10])
  rcybvt : Subsystem  mask(2-D Table){y=cybvtx_FMACH, z=cybvty_FALPHA, tab=cybvt}
      mask prompts: y "Y vector:"; z "Z vector:"; tab "Table:"
      mask help: 2-D Table Look Up. Enter monotonic Y and Z vectors and a matrix of 2-D tables. See the help for more info.
      mask Help: The Y and Z vectors must be monotonic.  Y  indexes into the columns of the 2-D table & Z indexes into the rows of the 2-D tables.   The input values are y and z respectively (e.g., top port = y).
      mask Display: plot(-10,-10,110,110,[90,50,10],[90,40,30],[90,50,10],[50,26,20],[90,50,10],[22,13,10])
  rcypwb : Subsystem  mask(2-D Table){y=cypwbx_FMACH, z=cypwby_FALPHA, tab=cypwb}
      mask prompts: y "Y vector:"; z "Z vector:"; tab "Table:"
      mask help: 2-D Table Look Up. Enter monotonic Y and Z vectors and a matrix of 2-D tables. See the help for more info.
      mask Help: The Y and Z vectors must be monotonic.  Y  indexes into the columns of the 2-D table & Z indexes into the rows of the 2-D tables.   The input values are y and z respectively (e.g., top port = y).
      mask Display: plot(-10,-10,110,110,[90,50,10],[90,40,30],[90,50,10],[50,26,20],[90,50,10],[22,13,10])
  dcyphat : Outport  OutDataType=sfix(16)  OutScaling=2^0  InitialOutput=0
  wires:
  constant3/1 -> Product2/1
  Product2/1 -> cyptail/1
  Switch7/1 -> cyptail/2, cypwb/2
  cypwb/1 -> cyptot/2
  rcypwb/1(Interp Value) -> cypwb/1
  CYPFLEX/1(cypfr) -> Switch7/1
  constant/1 -> Switch7/3
  rcybvt/1(Interp Value) -> Product2/5, Fcn28/1
  Fcn28/1 -> Product2/3
  rcrbvt/1(Interp Value) -> Product2/2
  alpha/1 -> rcrbvt/2(Z), rcybvt/2(Z), rcypwb/2(Z)
  altitude/1 -> CYPFLEX/1(altitude)
  flex/1 -> CYPFLEX/Enable, Switch7/2
  mach/1 -> rcrbvt/1(Y), rcybvt/1(Y), CYPFLEX/2(Mach), rcypwb/1(Y)
  constant2/1 -> Product2/4
  cyptail/1 -> cyptot/1
  p_prime/1 -> dcyrt/2
  cyptot/1 -> dcyrt/1
  dcyrt/1 -> dcyphat/1

== system gtm_aeromodel/get aero forces and moments/AERODYNAMICS/Force  Coefficients/SIDE/CYR ==
  mach : Inport  OutDataType=sfix(16)  OutScaling=2^0
  alpha : Inport  Port=2  OutDataType=sfix(16)  OutScaling=2^0
  altitude : Inport  Port=3  OutDataType=sfix(16)  OutScaling=2^0
  flex : Inport  Port=4  OutDataType=sfix(16)  OutScaling=2^0
  r_prime : Inport  Port=5  OutDataType=sfix(16)  OutScaling=2^0
  CYRFLEX : Subsystem  TreatAsAtomicUnit=on
  Fcn28 : Fcn  Expr=1/u
  Product2 : Product  Inputs=5  OutDataType=sfix(16)  OutScaling=2^0  SaturateOnIntegerOverflow=on  RndMeth=Zero  InputSameDT=on  OutDataTypeStr=Inherit: Same as first input
  Switch7 : Switch  Threshold=0.5  SaturateOnIntegerOverflow=on  InputSameDT=on
  cnbvt : Subsystem  mask(2-D Table){y=cnbvtx_FMACH, z=cnbvty_FALPHA, tab=cnbvt}
      mask prompts: y "Y vector:"; z "Z vector:"; tab "Table:"
      mask help: 2-D Table Look Up. Enter monotonic Y and Z vectors and a matrix of 2-D tables. See the help for more info.
      mask Help: The Y and Z vectors must be monotonic.  Y  indexes into the columns of the 2-D table & Z indexes into the rows of the 2-D tables.   The input values are y and z respectively (e.g., top port = y).
      mask Display: plot(-10,-10,110,110,[90,50,10],[90,40,30],[90,50,10],[50,26,20],[90,50,10],[22,13,10])
  constant : Constant  OutDataType=sfix(16)  OutScaling=2^0
  constant2 : Constant  Value=2  OutDataType=sfix(16)  OutScaling=2^0
  constant3 : Constant  Value=constants.r2d  OutDataType=sfix(16)  OutScaling=2^0
  cybvt : Subsystem  mask(2-D Table){y=cybvtx_FMACH, z=cybvty_FALPHA, tab=cybvt}
      mask prompts: y "Y vector:"; z "Z vector:"; tab "Table:"
      mask help: 2-D Table Look Up. Enter monotonic Y and Z vectors and a matrix of 2-D tables. See the help for more info.
      mask Help: The Y and Z vectors must be monotonic.  Y  indexes into the columns of the 2-D table & Z indexes into the rows of the 2-D tables.   The input values are y and z respectively (e.g., top port = y).
      mask Display: plot(-10,-10,110,110,[90,50,10],[90,40,30],[90,50,10],[50,26,20],[90,50,10],[22,13,10])
  cyrtail : Product  OutDataType=sfix(16)  OutScaling=2^0  SaturateOnIntegerOverflow=on  RndMeth=Zero  InputSameDT=on  OutDataTypeStr=Inherit: Same as first input
  cyrtot : Sum  Inputs=|++  OutDataType=sfix(16)  OutScaling=2^0  SaturateOnIntegerOverflow=on  InputSameDT=on  OutDataTypeStr=Inherit: Same as first input
  cyrwb : Product  OutDataType=sfix(16)  OutScaling=2^0  SaturateOnIntegerOverflow=on  RndMeth=Zero  InputSameDT=on  OutDataTypeStr=Inherit: Same as first input
  dcyrt : Product  OutDataType=sfix(16)  OutScaling=2^0  SaturateOnIntegerOverflow=on  RndMeth=Zero  InputSameDT=on  OutDataTypeStr=Inherit: Same as first input
  rcyrwb : Subsystem  mask(1-D Table){z=cyrwbx_FMACH, tab=cyrwb}
      mask prompts: z "Z vector:"; tab "Table:"
      mask help: 1-D Table Look Up. Enter monotonic Z vector amd table. See the help for more info.
      mask Help: The Z vector must be monotonic.  Z indexes into the columns of the 1-D tables.   Table does not extrapolate beyound the break vectors
      mask Display: plot(@2)
  dcyrhat : Outport  OutDataType=sfix(16)  OutScaling=2^0  InitialOutput=0
  wires:
  cybvt/1(Interp Value) -> Product2/5, Fcn28/1
  constant3/1 -> Product2/1
  cyrwb/1 -> cyrtot/2
  Switch7/1 -> cyrwb/2, cyrtail/2
  rcyrwb/1(Interp Value) -> cyrwb/1
  Product2/1 -> cyrtail/1
  CYRFLEX/1(cyrfr) -> Switch7/1
  constant/1 -> Switch7/3
  dcyrt/1 -> dcyrhat/1
  cyrtot/1 -> dcyrt/1
  r_prime/1 -> dcyrt/2
  cyrtail/1 -> cyrtot/1
  constant2/1 -> Product2/4
  mach/1 -> rcyrwb/1(Z), CYRFLEX/2(Mach), cybvt/1(Y), cnbvt/1(Y)
  flex/1 -> Switch7/2, CYRFLEX/Enable
  altitude/1 -> CYRFLEX/1(altitude)
  alpha/1 -> cybvt/2(Z), cnbvt/2(Z)
  cnbvt/1(Interp Value) -> Product2/2
  Fcn28/1 -> Product2/3

== system gtm_aeromodel/get aero forces and moments/AERODYNAMICS/Force  Coefficients/SIDE/CYRUD ==
  mach : Inport  OutDataType=sfix(16)  OutScaling=2^0
  rud : Inport  Port=2  OutDataType=sfix(16)  OutScaling=2^0
  altitude : Inport  Port=3  OutDataType=sfix(16)  OutScaling=2^0
  flex : Inport  Port=4  OutDataType=sfix(16)  OutScaling=2^0
  CYRFLEX : Subsystem  TreatAsAtomicUnit=on
  Product : Product  Inputs=3  OutDataType=sfix(16)  OutScaling=2^0  SaturateOnIntegerOverflow=on  RndMeth=Zero  InputSameDT=on  OutDataTypeStr=Inherit: Same as first input
  Switch7 : Switch  Threshold=0.5  SaturateOnIntegerOverflow=on  InputSameDT=on
  constant : Constant  OutDataType=sfix(16)  OutScaling=2^0
  cydr : Subsystem  mask(1-D Table){z=cydrx_FMACH, tab=cydr}
      mask prompts: z "Z vector:"; tab "Table:"
      mask help: 1-D Table Look Up. Enter monotonic Z vector amd table. See the help for more info.
      mask Help: The Z vector must be monotonic.  Z indexes into the columns of the 1-D tables.   Table does not extrapolate beyound the break vectors
      mask Display: plot(@2)
  cyrud : Outport  OutDataType=sfix(16)  OutScaling=2^0  InitialOutput=0
  wires:
  constant/1 -> Switch7/3
  CYRFLEX/1(cyrfr) -> Switch7/1
  flex/1 -> Switch7/2, CYRFLEX/Enable
  Switch7/1 -> Product/3
  Product/1 -> cyrud/1
  mach/1 -> CYRFLEX/2(Mach), cydr/1(Z)
  altitude/1 -> CYRFLEX/1(altitude)
  rud/1 -> Product/2
  cydr/1(Interp Value) -> Product/1
